simulink model "Final_Delta_Simscape_4"  (R2023a)
settings: Solver=FixedStepAuto  StartTime=0.0  StopTime=10.0  FixedStep=0.01  RelTol=1e-3
model workspace: external: MATLAB File D:\TAI LIEU MON HOC\Do_an_tot_nghiep\Simscape\Final_Delta_Simscape_4_DataFile.m (data not in the file)
undefined symbols (not defined in the file or in its folder): smiData, X, Y, Z
libraries: sm_lib x272, nesl_utility x19, simulink_extras x6
(part 6 of 6)

== system Final_Delta_Simscape_4/Subsystem/SubTayDuoi_6_RIGID/Ball_Washer_HS_2_RIGID ==
  ReferenceFrame : sm_lib/Frames and Transforms/Reference Frame
  Solid : sm_lib/Body Elements/File Solid  ExtGeomFileName=Ball Washer HS_Default_sldprt.STEP  UnitType=FromFile  ExtGeomFileUnits=m  StepReaderType=HEX  ExportConvexHullGeometry=off  InertiaType=Custom  Mass=smiData.Solid(3).mass  MassUnits=kg  CenterOfMass=smiData.Solid(3).CoM  CenterOfMassUnits=mm  MomentsOfInertia=smiData.Solid(3).MoI  MomentsOfInertiaUnits=kg*mm^2  ProductsOfInertia=smiData.Solid(3).PoI  ProductsOfInertiaUnits=kg*mm^2  BasedOnType=DensityFromFile  Density=1000  DensityUnits=kg/m^3  DoExposeReferenceFrame=on  SerializedFrames=<Frames/>  GraphicType=FromGeometry  MarkerShape=Sphere  MarkerSize=10  GraphicVisPropType=SimpleVisualProperties  GraphicDiffuseColor=smiData.Solid(3).color  GraphicSpecularColor=[0.5 0.5 0.5 1.0]  GraphicAmbientColor=[0.15 0.15 0.15 1.0]  GraphicEmissiveColor=[0.0 0.0 0.0 1.0]  GraphicShininess=75  GraphicOpacity=smiData.Solid(3).opacity
  F : PMIOPort  Side=Left
  connections:
  Solid/RConn1 -- ReferenceFrame/RConn1 -- F/RConn1

== system Final_Delta_Simscape_4/Subsystem/SubTayDuoi_6_RIGID/Male_Rod_End_Bearing_HS_1_RIGID ==
  ReferenceFrame : sm_lib/Frames and Transforms/Reference Frame
  Solid : sm_lib/Body Elements/File Solid  ExtGeomFileName=Male Rod End Bearing HS_Default_sldprt.STEP  UnitType=FromFile  ExtGeomFileUnits=m  StepReaderType=HEX  ExportConvexHullGeometry=off  InertiaType=Custom  Mass=smiData.Solid(2).mass  MassUnits=kg  CenterOfMass=smiData.Solid(2).CoM  CenterOfMassUnits=mm  MomentsOfInertia=smiData.Solid(2).MoI  MomentsOfInertiaUnits=kg*mm^2  ProductsOfInertia=smiData.Solid(2).PoI  ProductsOfInertiaUnits=kg*mm^2  BasedOnType=DensityFromFile  Density=1000  DensityUnits=kg/m^3  DoExposeReferenceFrame=on  SerializedFrames=<Frames/>  GraphicType=FromGeometry  MarkerShape=Sphere  MarkerSize=10  GraphicVisPropType=SimpleVisualProperties  GraphicDiffuseColor=smiData.Solid(2).color  GraphicSpecularColor=[0.5 0.5 0.5 1.0]  GraphicAmbientColor=[0.15 0.15 0.15 1.0]  GraphicEmissiveColor=[0.0 0.0 0.0 1.0]  GraphicShininess=75  GraphicOpacity=smiData.Solid(2).opacity
  F : PMIOPort  Side=Left
  connections:
  Solid/RConn1 -- ReferenceFrame/RConn1 -- F/RConn1

== system Final_Delta_Simscape_4/Subsystem/SubTayDuoi_6_RIGID/Male_Rod_End_Bearing_HS_2_RIGID ==
  ReferenceFrame : sm_lib/Frames and Transforms/Reference Frame
  Solid : sm_lib/Body Elements/File Solid  ExtGeomFileName=Male Rod End Bearing HS_Default_sldprt.STEP  UnitType=FromFile  ExtGeomFileUnits=m  StepReaderType=HEX  ExportConvexHullGeometry=off  InertiaType=Custom  Mass=smiData.Solid(2).mass  MassUnits=kg  CenterOfMass=smiData.Solid(2).CoM  CenterOfMassUnits=mm  MomentsOfInertia=smiData.Solid(2).MoI  MomentsOfInertiaUnits=kg*mm^2  ProductsOfInertia=smiData.Solid(2).PoI  ProductsOfInertiaUnits=kg*mm^2  BasedOnType=DensityFromFile  Density=1000  DensityUnits=kg/m^3  DoExposeReferenceFrame=on  SerializedFrames=<Frames/>  GraphicType=FromGeometry  MarkerShape=Sphere  MarkerSize=10  GraphicVisPropType=SimpleVisualProperties  GraphicDiffuseColor=smiData.Solid(2).color  GraphicSpecularColor=[0.5 0.5 0.5 1.0]  GraphicAmbientColor=[0.15 0.15 0.15 1.0]  GraphicEmissiveColor=[0.0 0.0 0.0 1.0]  GraphicShininess=75  GraphicOpacity=smiData.Solid(2).opacity
  F : PMIOPort  Side=Left
  connections:
  Solid/RConn1 -- ReferenceFrame/RConn1 -- F/RConn1

== system Final_Delta_Simscape_4/Subsystem/SubTayDuoi_6_RIGID/TayDuoi_1_RIGID ==
  ReferenceFrame : sm_lib/Frames and Transforms/Reference Frame
  Solid : sm_lib/Body Elements/File Solid  ExtGeomFileName=TayDuoi_Default_sldprt.STEP  UnitType=FromFile  ExtGeomFileUnits=m  StepReaderType=HEX  ExportConvexHullGeometry=off  InertiaType=Custom  Mass=smiData.Solid(1).mass  MassUnits=kg  CenterOfMass=smiData.Solid(1).CoM  CenterOfMassUnits=mm  MomentsOfInertia=smiData.Solid(1).MoI  MomentsOfInertiaUnits=kg*mm^2  ProductsOfInertia=smiData.Solid(1).PoI  ProductsOfInertiaUnits=kg*mm^2  BasedOnType=DensityFromFile  Density=1000  DensityUnits=kg/m^3  DoExposeReferenceFrame=on  SerializedFrames=<Frames/>  GraphicType=FromGeometry  MarkerShape=Sphere  MarkerSize=10  GraphicVisPropType=SimpleVisualProperties  GraphicDiffuseColor=smiData.Solid(1).color  GraphicSpecularColor=[0.5 0.5 0.5 1.0]  GraphicAmbientColor=[0.15 0.15 0.15 1.0]  GraphicEmissiveColor=[0.0 0.0 0.0 1.0]  GraphicShininess=75  GraphicOpacity=smiData.Solid(1).opacity
  F : PMIOPort  Side=Left
  connections:
  Solid/RConn1 -- ReferenceFrame/RConn1 -- F/RConn1

== system Final_Delta_Simscape_4/Subsystem/Top_Delta_Simscape_1_RIGID/BaseA_Simscape_1_RIGID ==
  ReferenceFrame : sm_lib/Frames and Transforms/Reference Frame
  Solid : sm_lib/Body Elements/File Solid  ExtGeomFileName=BaseA_Simscape_Default_sldprt.STEP  UnitType=FromFile  ExtGeomFileUnits=m  StepReaderType=HEX  ExportConvexHullGeometry=off  InertiaType=Custom  Mass=smiData.Solid(9).mass  MassUnits=kg  CenterOfMass=smiData.Solid(9).CoM  CenterOfMassUnits=mm  MomentsOfInertia=smiData.Solid(9).MoI  MomentsOfInertiaUnits=kg*mm^2  ProductsOfInertia=smiData.Solid(9).PoI  ProductsOfInertiaUnits=kg*mm^2  BasedOnType=DensityFromFile  Density=1000  DensityUnits=kg/m^3  DoExposeReferenceFrame=on  SerializedFrames=<Frames/>  GraphicType=FromGeometry  MarkerShape=Sphere  MarkerSize=10  GraphicVisPropType=SimpleVisualProperties  GraphicDiffuseColor=smiData.Solid(9).color  GraphicSpecularColor=[0.5 0.5 0.5 1.0]  GraphicAmbientColor=[0.15 0.15 0.15 1.0]  GraphicEmissiveColor=[0.0 0.0 0.0 1.0]  GraphicShininess=75  GraphicOpacity=smiData.Solid(9).opacity
  F : PMIOPort  Side=Left
  connections:
  Solid/RConn1 -- ReferenceFrame/RConn1 -- F/RConn1

== system Final_Delta_Simscape_4/Subsystem/Top_Delta_Simscape_1_RIGID/Fake_Motor_1_RIGID ==
  ReferenceFrame : sm_lib/Frames and Transforms/Reference Frame
  Solid : sm_lib/Body Elements/File Solid  ExtGeomFileName=Fake Motor_Default_sldprt.STEP  UnitType=FromFile  ExtGeomFileUnits=m  StepReaderType=HEX  ExportConvexHullGeometry=off  InertiaType=Custom  Mass=smiData.Solid(7).mass  MassUnits=kg  CenterOfMass=smiData.Solid(7).CoM  CenterOfMassUnits=mm  MomentsOfInertia=smiData.Solid(7).MoI  MomentsOfInertiaUnits=kg*mm^2  ProductsOfInertia=smiData.Solid(7).PoI  ProductsOfInertiaUnits=kg*mm^2  BasedOnType=DensityFromFile  Density=1000  DensityUnits=kg/m^3  DoExposeReferenceFrame=on  SerializedFrames=<Frames/>  GraphicType=FromGeometry  MarkerShape=Sphere  MarkerSize=10  GraphicVisPropType=SimpleVisualProperties  GraphicDiffuseColor=smiData.Solid(7).color  GraphicSpecularColor=[0.5 0.5 0.5 1.0]  GraphicAmbientColor=[0.15 0.15 0.15 1.0]  GraphicEmissiveColor=[0.0 0.0 0.0 1.0]  GraphicShininess=75  GraphicOpacity=smiData.Solid(7).opacity
  F : PMIOPort  Side=Left
  connections:
  Solid/RConn1 -- ReferenceFrame/RConn1 -- F/RConn1

== system Final_Delta_Simscape_4/Subsystem/Top_Delta_Simscape_1_RIGID/Fake_Motor_2_RIGID ==
  ReferenceFrame : sm_lib/Frames and Transforms/Reference Frame
  Solid : sm_lib/Body Elements/File Solid  ExtGeomFileName=Fake Motor_Default_sldprt.STEP  UnitType=FromFile  ExtGeomFileUnits=m  StepReaderType=HEX  ExportConvexHullGeometry=off  InertiaType=Custom  Mass=smiData.Solid(7).mass  MassUnits=kg  CenterOfMass=smiData.Solid(7).CoM  CenterOfMassUnits=mm  MomentsOfInertia=smiData.Solid(7).MoI  MomentsOfInertiaUnits=kg*mm^2  ProductsOfInertia=smiData.Solid(7).PoI  ProductsOfInertiaUnits=kg*mm^2  BasedOnType=DensityFromFile  Density=1000  DensityUnits=kg/m^3  DoExposeReferenceFrame=on  SerializedFrames=<Frames/>  GraphicType=FromGeometry  MarkerShape=Sphere  MarkerSize=10  GraphicVisPropType=SimpleVisualProperties  GraphicDiffuseColor=smiData.Solid(7).color  GraphicSpecularColor=[0.5 0.5 0.5 1.0]  GraphicAmbientColor=[0.15 0.15 0.15 1.0]  GraphicEmissiveColor=[0.0 0.0 0.0 1.0]  GraphicShininess=75  GraphicOpacity=smiData.Solid(7).opacity
  F : PMIOPort  Side=Left
  connections:
  Solid/RConn1 -- ReferenceFrame/RConn1 -- F/RConn1

== system Final_Delta_Simscape_4/Subsystem/Top_Delta_Simscape_1_RIGID/Fake_Motor_3_RIGID ==
  ReferenceFrame : sm_lib/Frames and Transforms/Reference Frame
  Solid : sm_lib/Body Elements/File Solid  ExtGeomFileName=Fake Motor_Default_sldprt.STEP  UnitType=FromFile  ExtGeomFileUnits=m  StepReaderType=HEX  ExportConvexHullGeometry=off  InertiaType=Custom  Mass=smiData.Solid(7).mass  MassUnits=kg  CenterOfMass=smiData.Solid(7).CoM  CenterOfMassUnits=mm  MomentsOfInertia=smiData.Solid(7).MoI  MomentsOfInertiaUnits=kg*mm^2  ProductsOfInertia=smiData.Solid(7).PoI  ProductsOfInertiaUnits=kg*mm^2  BasedOnType=DensityFromFile  Density=1000  DensityUnits=kg/m^3  DoExposeReferenceFrame=on  SerializedFrames=<Frames/>  GraphicType=FromGeometry  MarkerShape=Sphere  MarkerSize=10  GraphicVisPropType=SimpleVisualProperties  GraphicDiffuseColor=smiData.Solid(7).color  GraphicSpecularColor=[0.5 0.5 0.5 1.0]  GraphicAmbientColor=[0.15 0.15 0.15 1.0]  GraphicEmissiveColor=[0.0 0.0 0.0 1.0]  GraphicShininess=75  GraphicOpacity=smiData.Solid(7).opacity
  F : PMIOPort  Side=Left
  connections:
  Solid/RConn1 -- ReferenceFrame/RConn1 -- F/RConn1

== system Final_Delta_Simscape_4/Subsystem/Top_Delta_Simscape_1_RIGID/PartARM_4_RIGID ==
  ReferenceFrame : sm_lib/Frames and Transforms/Reference Frame
  Solid : sm_lib/Body Elements/File Solid  ExtGeomFileName=PartARM_Default_sldprt.STEP  UnitType=FromFile  ExtGeomFileUnits=m  StepReaderType=HEX  ExportConvexHullGeometry=off  InertiaType=Custom  Mass=smiData.Solid(8).mass  MassUnits=kg  CenterOfMass=smiData.Solid(8).CoM  CenterOfMassUnits=mm  MomentsOfInertia=smiData.Solid(8).MoI  MomentsOfInertiaUnits=kg*mm^2  ProductsOfInertia=smiData.Solid(8).PoI  ProductsOfInertiaUnits=kg*mm^2  BasedOnType=DensityFromFile  Density=1000  DensityUnits=kg/m^3  DoExposeReferenceFrame=on  SerializedFrames=<Frames/>  GraphicType=FromGeometry  MarkerShape=Sphere  MarkerSize=10  GraphicVisPropType=SimpleVisualProperties  GraphicDiffuseColor=smiData.Solid(8).color  GraphicSpecularColor=[0.5 0.5 0.5 1.0]  GraphicAmbientColor=[0.15 0.15 0.15 1.0]  GraphicEmissiveColor=[0.0 0.0 0.0 1.0]  GraphicShininess=75  GraphicOpacity=smiData.Solid(8).opacity
  F : PMIOPort  Side=Left
  connections:
  Solid/RConn1 -- ReferenceFrame/RConn1 -- F/RConn1

== system Final_Delta_Simscape_4/Subsystem/Top_Delta_Simscape_1_RIGID/PartARM_5_RIGID ==
  ReferenceFrame : sm_lib/Frames and Transforms/Reference Frame
  Solid : sm_lib/Body Elements/File Solid  ExtGeomFileName=PartARM_Default_sldprt.STEP  UnitType=FromFile  ExtGeomFileUnits=m  StepReaderType=HEX  ExportConvexHullGeometry=off  InertiaType=Custom  Mass=smiData.Solid(8).mass  MassUnits=kg  CenterOfMass=smiData.Solid(8).CoM  CenterOfMassUnits=mm  MomentsOfInertia=smiData.Solid(8).MoI  MomentsOfInertiaUnits=kg*mm^2  ProductsOfInertia=smiData.Solid(8).PoI  ProductsOfInertiaUnits=kg*mm^2  BasedOnType=DensityFromFile  Density=1000  DensityUnits=kg/m^3  DoExposeReferenceFrame=on  SerializedFrames=<Frames/>  GraphicType=FromGeometry  MarkerShape=Sphere  MarkerSize=10  GraphicVisPropType=SimpleVisualProperties  GraphicDiffuseColor=smiData.Solid(8).color  GraphicSpecularColor=[0.5 0.5 0.5 1.0]  GraphicAmbientColor=[0.15 0.15 0.15 1.0]  GraphicEmissiveColor=[0.0 0.0 0.0 1.0]  GraphicShininess=75  GraphicOpacity=smiData.Solid(8).opacity
  F : PMIOPort  Side=Left
  connections:
  Solid/RConn1 -- ReferenceFrame/RConn1 -- F/RConn1

== system Final_Delta_Simscape_4/Subsystem/Top_Delta_Simscape_1_RIGID/PartARM_6_RIGID ==
  ReferenceFrame : sm_lib/Frames and Transforms/Reference Frame
  Solid : sm_lib/Body Elements/File Solid  ExtGeomFileName=PartARM_Default_sldprt.STEP  UnitType=FromFile  ExtGeomFileUnits=m  StepReaderType=HEX  ExportConvexHullGeometry=off  InertiaType=Custom  Mass=smiData.Solid(8).mass  MassUnits=kg  CenterOfMass=smiData.Solid(8).CoM  CenterOfMassUnits=mm  MomentsOfInertia=smiData.Solid(8).MoI  MomentsOfInertiaUnits=kg*mm^2  ProductsOfInertia=smiData.Solid(8).PoI  ProductsOfInertiaUnits=kg*mm^2  BasedOnType=DensityFromFile  Density=1000  DensityUnits=kg/m^3  DoExposeReferenceFrame=on  SerializedFrames=<Frames/>  GraphicType=FromGeometry  MarkerShape=Sphere  MarkerSize=10  GraphicVisPropType=SimpleVisualProperties  GraphicDiffuseColor=smiData.Solid(8).color  GraphicSpecularColor=[0.5 0.5 0.5 1.0]  GraphicAmbientColor=[0.15 0.15 0.15 1.0]  GraphicEmissiveColor=[0.0 0.0 0.0 1.0]  GraphicShininess=75  GraphicOpacity=smiData.Solid(8).opacity
  F : PMIOPort  Side=Left
  connections:
  Solid/RConn1 -- ReferenceFrame/RConn1 -- F/RConn1

== matlab function Final_Delta_Simscape_4/MATLAB Function1 ==
  data: X_ee input; theta1 output; Y_ee input; Z_ee input; theta2 output; theta3 output
function [theta1, theta2, theta3] = Inverse_Kinamatic(X_ee,Y_ee,Z_ee)
    R_Base = 60;
    R_platform = 42.62; % Khoảng cách từ tâm end_effector tới khớp cầu
    r = R_Base - R_platform;   % Khoảng cách từ tâm top tới động cơ
    
    re = 150;       % Chiều dài cánh tay trên (mm)
    rf = 350;       % Chiều dài cánh tay dưới (mm)
    % Z_ee = Z_ee+35.5;
    % Góc xoay động cơ 
    alpha = [0, 120, 240] * pi / 180;
    
    J = zeros(3, 1);
    threshold = 1e-3;
    for i = 1:3
        A = -2*re*(-r+X_ee*cos(alpha(i))+Y_ee*sin(alpha(i)));
        B = -2*re*Z_ee;
        C = X_ee^2 + Y_ee^2 + Z_ee^2 + r^2 + re^2 - rf^2 - 2*r*(X_ee*cos(alpha(i))+Y_ee*sin(alpha(i)));
        ABC = [A;B;C];
        theta_1 = atan2(B,A) + acos(-C/sqrt((A)^2+(B)^2));
        theta_2 = atan2(B,A) - acos(-C/sqrt((A)^2+(B)^2));
        if theta_1 > theta_2
            theta = theta_2;
        else theta = theta_1;
        end
        % Kiểm tra nếu góc quá nhỏ, đặt theta = 0
        if abs(theta) < threshold
            theta = 0;
        end
        theta = theta*180/pi;
        J(i,1) = -theta;
    end
   % K = J(:,:)
   theta1 = J(1);
   theta2 = J(2);
   theta3 = J(3);
end

== matlab function Final_Delta_Simscape_4/MATLAB Function ==
  data: theta1 input; Px output; theta2 input; theta3 input; Py output; Pz output
function [Px,Py,Pz] = Forward_Kinamatic(theta1, theta2, theta3)
    % Các thông số hình học của robot Delta

    R_Base = 60 ;  % Khoảng cách từ tâm top tới động cơ
    R_platform = 42.62; % Khoảng cách từ tâm end_effector tới khớp cầu
    r = R_Base-R_platform;

    re = 150;       % Chiều dài cánh tay trên (mm)
    rf = 350;       % Chiều dài cánh tay dưới (mm)
    theta_in = [theta1, theta2, theta3] * pi / 180;
    
    % Góc xoay động cơ 
    alpha_base = [0, 120, 240] * pi / 180;
    
    % Tính toán vị trí của các khớp di động
    P = zeros(3, 3);
    for i = 1:3
        Px = r + re * cos(theta_in(i));
        Py = 0;
        Pz = -re * sin(theta_in(i));
        K = [Px; Py; Pz];
        P(i, :) = Rz(alpha_base(i)) * K;
    end
    P_Original = P;
    P_origin = -P(1, 1:3)';

    motor_positions = zeros(3,3);
    for i = 1:3
        motor_positions(i,1) = P_origin(1) + (r+R_platform) * cos(alpha_base(i));
        motor_positions(i,2) = P_origin(2) + (r+R_platform) * sin(alpha_base(i));
        motor_positions(i,3) = P_origin(3); % Động cơ nằm trên cùng một mặt phẳng
    end   
    
    % Đặt J1 làm gốc tọa độ
    P = P - P(1, :);

    % Tính toán hệ trục tọa độ
    J1_J3 = [P(3,1)-P(1,1); P(3,2)-P(1,2); P(3,3)-P(1,3)];
    J3_J1 = [P(1,1)-P(3,1); P(1,2)-P(3,2); P(1,3)-P(3,3)];
    J1_J2 = [P(2,1)-P(1,1); P(2,2)-P(1,2); P(2,3)-P(1,3)];
    
    ex_hat = J1_J2 / norm(J1_J2);
    a = dot(ex_hat, J1_J3);
    ey_hat = (J3_J1 + a * ex_hat) / norm(J3_J1 + a * ex_hat);
    % ey_hat = [(J3_J1(1)+a*ex_hat(1))/sqrt((J3_J1(1)+a*ex_hat(1))^2+(J3_J1(2)+a*ex_hat(2))^2) ; ...
    %            (J3_J1(2)+a*ex_hat(2))/sqrt((J3_J1(1)+a*ex_hat(1))^2+(J3_J1(2)+a*ex_hat(2))^2);0]
    ez_hat = cross(ex_hat, ey_hat);
    
    % Tính toán vị trí end-effector
    b = dot(ey_hat, J1_J3);
    d = norm(J1_J2);
    x = d / 2;
    y = (a^2 + b^2) / (2*b) - a*x/b;
    z = sqrt(rf^2 - x^2 - y^2);
    
    % end_effector = x * ex_hat + y * ey_hat + z * ez_hat
    P_0_ee = [P_Original(1)+x*ex_hat(1)+y*ey_hat(1)+z*ez_hat(1);...
                    P_Original(1,2)+x*ex_hat(2)+y*ey_hat(2)+z*ez_hat(2);...
                    P_Original(1,3)+x*ex_hat(3)+y*ey_hat(3)+z*ez_hat(3)];

    P_J1_ee = P_0_ee + P_origin;
    % P_0_ee = P_J1_e - P_origin;
    Px = P_0_ee(1);
    Py = P_0_ee(2);
    Pz = P_0_ee(3);

end

function R = Rz(q)
R=[cos(q) -sin(q) 0 
    sin(q) cos(q) 0;
    0 0 1];
end

function T = Rotz(q)
R=Rz(q);
T=[R(1,1) R(1,2) R(1,3) 0;
   R(2,1) R(2,2) R(2,3) 0;
   R(3,1) R(3,2) R(3,3) 0;
   0 0 0 1];
end

== matlab function Final_Delta_Simscape_4/MATLAB Function2 ==
  data: x output; t input; y output; P0 input; v0 input; a0 input; t0 input; Pf input; vf input; af input; tf input; z output
function [x,y,z] = TrajectoryPlanning_2_point(t,P0,v0,a0,t0,Pf,vf,af,tf)

xA = P0(1);
xA_velocity = v0(1);
xA_accelerate = a0(1);
xB = Pf(1);
xB_velocity = vf(1);
xB_accelerate = af(1);


yA = P0(2);
yA_velocity = v0(2);
yA_accelerate = a0(2);
yB = Pf(2);
yB_velocity = vf(2);
yB_accelerate = af(2);

zA = P0(3);
zA_velocity = v0(3);
zA_accelerate = a0(3);
zB = Pf(3);
zB_velocity = vf(3);
zB_accelerate = af(3);

% B = [1,t0,t0^2,t0^3;0,1,2*t0,3*t0^2;1,tf,tf^2,tf^3;0,1,2*tf,3*tf^2];
B = [1,t0,t0^2,t0^3,t0^4,t0^5;...
     0,1,2*t0,3*t0^2,4*t0^3,5*t0^4;...
     0,0,2,6*t0,12*t0^2,20*t0^3;...
     1,tf,tf^2,tf^3,tf^4,tf^5;...
     0,1,2*tf,3*tf^2,4*tf^3,5*tf^4;...
     0,0,2,6*tf,12*tf^2,20*tf^3];
invB = inv(B);

result_1 = invB*[xA;xA_velocity;xA_accelerate;xB;xB_velocity;xB_accelerate];
result_2 = invB*[yA;yA_velocity;yA_accelerate;yB;yB_velocity;yB_accelerate];
result_3 = invB*[zA;zA_velocity;zA_accelerate;zB;zB_velocity;zB_accelerate];

if t<t0
     x=P0(1);
     y=P0(2);  
     z=P0(3);
elseif t<=tf    
     a10 = result_1(1);
     a11 = result_1(2);
     a12 = result_1(3);
     a13 = result_1(4);
     a14 = result_1(5);
     a15 = result_1(6);
    
     a20 = result_2(1);
     a21 = result_2(2);
     a22 = result_2(3);
     a23 = result_2(4);
     a24 = result_2(5);
     a25 = result_2(6);

     a30 = result_3(1);
     a31 = result_3(2);
     a32 = result_3(3);
     a33 = result_3(4);
     a34 = result_3(5);
     a35 = result_3(6);
     tt= t;
     x = a10+a11*tt+a12*tt^2+a13*tt^3+a14*tt^4+a15*tt^5;
     y = a20+a21*tt+a22*tt^2+a23*tt^3+a24*tt^4+a25*tt^5;
     z = a30+a31*tt+a32*tt^2+a33*tt^3+a34*tt^4+a35*tt^5;
else
     x=Pf(1);
     y=Pf(2);
     z=Pf(3);
end
% hold on;
% plot3(x, y, z, 'bo'); % Vẽ điểm hiện tại
% xlabel('X-axis'); ylabel('Y-axis'); zlabel('Z-axis');
% grid on;
% view(3);
% drawnow;
end

== matlab function Final_Delta_Simscape_4/MATLAB Function3 ==
  data: x output; t input; y output; P0 input; t0 input; Pf input; tf input; z output
function [x,y,z] = TrajectoryPlanning_2_point(t, P0, t0, Pf, tf)

% Giả định: t0 = 0, v0 = vf = 0, a0 = af = 0
% => áp dụng công thức trajectory bậc 5 đơn giản

% Tính hệ số cho x
delta_x = Pf(1) - P0(1);
a0x = P0(1);
a1x = 0;
a2x = 0;
a3x = 10 * delta_x / tf^3;
a4x = -15 * delta_x / tf^4;
a5x = 6 * delta_x / tf^5;

% Tính hệ số cho y
delta_y = Pf(2) - P0(2);
a0y = P0(2);
a1y = 0;
a2y = 0;
a3y = 10 * delta_y / tf^3;
a4y = -15 * delta_y / tf^4;
a5y = 6 * delta_y / tf^5;

% Tính hệ số cho z
delta_z = Pf(3) - P0(3);
a0z = P0(3);
a1z = 0;
a2z = 0;
a3z = 10 * delta_z / tf^3;
a4z = -15 * delta_z / tf^4;
a5z = 6 * delta_z / tf^5;

if t < t0
    x = P0(1);
    y = P0(2);
    z = P0(3);
elseif t <= tf
    x = a0x + a1x*t + a2x*t^2 + a3x*t^3 + a4x*t^4 + a5x*t^5;
    y = a0y + a1y*t + a2y*t^2 + a3y*t^3 + a4y*t^4 + a5y*t^5;
    z = a0z + a1z*t + a2z*t^2 + a3z*t^3 + a4z*t^4 + a5z*t^5;
else
    x = Pf(1);
    y = Pf(2);
    z = Pf(3);
end
hold on;
plot3(x, y, z, 'bo'); % Vẽ điểm hiện tại
xlabel('X-axis'); ylabel('Y-axis'); zlabel('Z-axis');
grid on;
view(3);
drawnow;

end
